simulink model "CSTR_Simulation"  (R2023a)
settings: Solver=VariableStepAuto  StartTime=0.0  StopTime=10.0  RelTol=1e-3
settings Model: Creator=rushs  LastModifiedBy=rushs

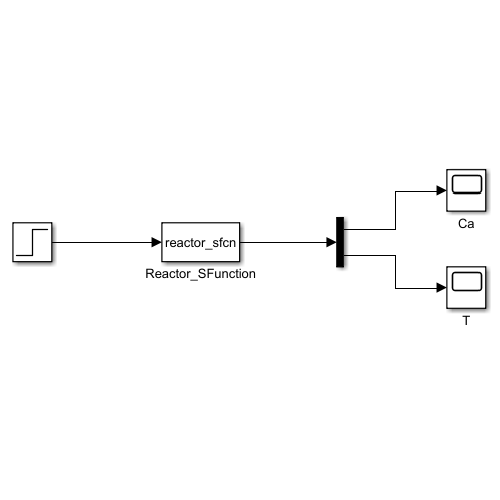
[thumbnail: Simulink's stored preview of the top-level diagram]
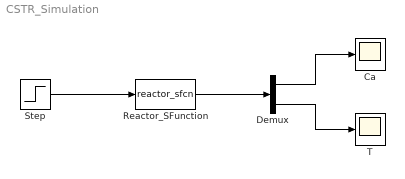
== system CSTR_Simulation ==
  Ca : Scope
  Demux : Demux  Outputs=2
  Reactor_SFunction : S-Function  FunctionName=reactor_sfcn  Parameters=0.1, 40  SFunctionDeploymentMode=off  EnableBusSupport=off
  Step : Step  SampleTime=0
  T : Scope
  wires:
  Step/1 -> Reactor_SFunction/1
  Reactor_SFunction/1 -> Demux/1
  Demux/1 -> Ca/1
  Demux/2 -> T/1
